simulink model "zhh"  (Simulink 7.9)
settings: Solver=FixedStepDiscrete  StartTime=0.0  StopTime=inf  FixedStep=1/256  MaxStep=1/256  RelTol=1e-3
undefined symbols (not defined in the file or in its folder): currentCFG_zhh_UB, UB
libraries: Tools x2, ScopeScaler x1, gUSBamplib x1
settings Model: Creator=gtec  LastModifiedBy=ECUSTBCI
settings OptimizationCC: InitFltsAndDblsToZero=on
settings DebuggingCC: MultiTaskCondExecSysMsg=none  FcnCallInpInsideContextMsg=Use local settings  FrameProcessingCompatibilityMsg=error  StrictBusMsg=Warning
settings GRTTargetCC: CombineOutputUpdateFcns=off  GRTInterface=on

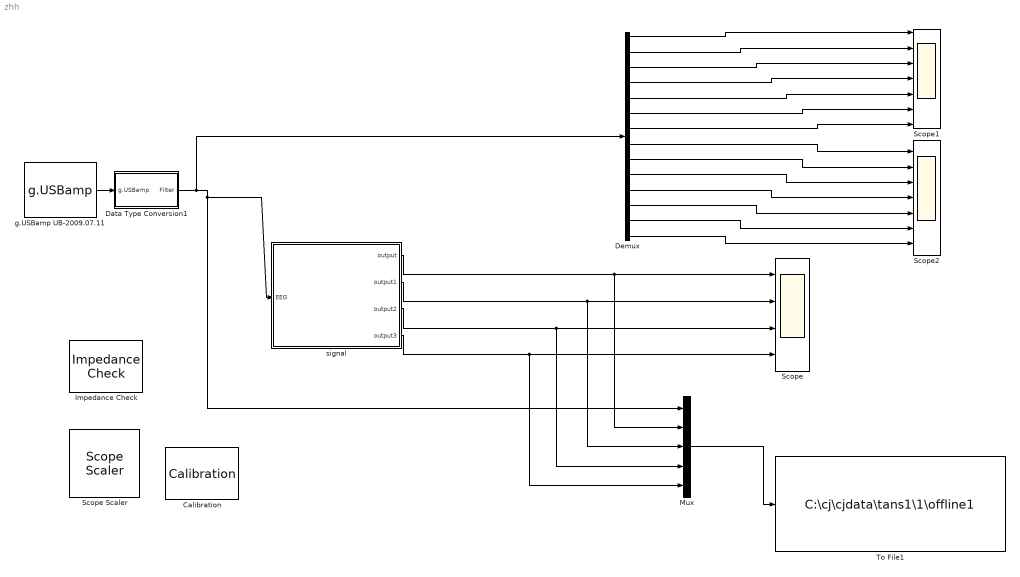
== system zhh ==
  Calibration : Tools/Calibration  SystemSampleTime=-1
  Data Type Conversion1 : Subsystem
  Demux : Demux  Outputs=14
  Impedance Check : Tools/Impedance Check  SystemSampleTime=-1
  Mux : Mux  Inputs=5
  Scope : Scope  NumInputPorts=4
      settings: TimeRange=10  YMin=9.5~9.5~9.5~9.5  YMax=10.5~10.5~10.5~10.5
  Scope Scaler : ScopeScaler/Scope Scaler  SystemSampleTime=-1
  Scope1 : Scope  NumInputPorts=7
      settings: TickLabels=off  TimeRange=10  YMin=-50~-50~-50~-50~-50~-50~-50  YMax=50~50~50~50~50~50~50  SampleTime=1/256
  Scope2 : Scope  NumInputPorts=7
      settings: TickLabels=off  TimeRange=10  YMin=-50~-50~-50~-50~-50~-50~-50  YMax=50~50~50~50~50~50~50  SaveName=ScopeData2  SampleTime=1/256
  To File1 : ToFile  Filename=C:\cj\cjdata\tans1\1\offline1  MatrixName=y
  g.USBamp UB-2009.07.11 : gUSBamplib/g.USBamp  Priority=2  cfg=currentCFG_zhh_UB-2009.07.11.cfg  snr=UB-2009.07.11
  signal : Subsystem  mask{host='192.168.1.3;192.168.1.103', socket='50000;31500', NumCustomCmds=12, ISI=500, SimNumTrials=20, ResetSpellerPeriod=300, PausePeriod=500, SampleRate=256, Determination=1, channels=14, selectchannles=[1:14], BaseAver=2, rep=2, targetp=[1 2 3 4 5 99 99 99 14 15 16 17 18 99 99 99 31 32 33 34 35 99 99 99 99 99  ], starget=1, traintime=3}
      mask prompts: host "P300host"; socket "P300socket"; NumCustomCmds "P300NumCustomCmds"; ISI "P300ISI"; SimNumTrials "P300SimNumTrials"; ResetSpellerPeriod "P300ResetSpellerPeriod"; PausePeriod "P300PausePeriod"; SampleRate "P300SampleRate"; Determination "P300Determination(classfier,yes,no)"; channels "Channles"; selectchannles "select Channels"; BaseAver "P300BaseAverage"; rep "P300reptimes"; targetp "P300target"; starget "s-target"
      mask Display:
      | image(imread('C:\tools\gtec\SSVEPP300_NET\SSVEP_MODEL2.tif'))
      | port_label('output', 1, 'flash')
      | port_label('output', 2, 'trial')
      | port_label('input', 1, 'EEG')
  wires:
  Data Type Conversion1/1(Filter) -> Mux/1, signal/1(EEG), Demux/1
  Mux/1 -> To File1/1
  signal/1(output) -> Scope/1, Mux/2
  signal/2(output1) -> Scope/2, Mux/3
  signal/3(output2) -> Scope/3, Mux/4
  signal/4(output3) -> Scope/4, Mux/5
  g.USBamp UB-2009.07.11/1 -> Data Type Conversion1/1(g.USBamp)
  Demux/1 -> Scope1/1
  Demux/2 -> Scope1/2
  Demux/3 -> Scope1/3
  Demux/4 -> Scope1/4
  Demux/5 -> Scope1/5
  Demux/6 -> Scope1/6
  Demux/7 -> Scope1/7
  Demux/8 -> Scope2/1
  Demux/9 -> Scope2/2
  Demux/10 -> Scope2/3
  Demux/11 -> Scope2/4
  Demux/12 -> Scope2/5
  Demux/13 -> Scope2/6
  Demux/14 -> Scope2/7

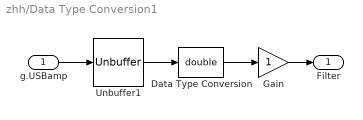
== system zhh/Data Type Conversion1 ==
  g.USBamp : Inport  Priority=1
  Data Type Conversion : DataTypeConversion  OutDataTypeStr=double
  Gain : Gain  SampleTime=1/256  SaturateOnIntegerOverflow=on  OutDataTypeStr=Inherit: Same as input  ParamDataTypeStr=Inherit: Same as input
  Unbuffer1 : Unbuffer  SampleBasedProcessing=Same as frame based
  Filter : Outport
  wires:
  Data Type Conversion/1 -> Gain/1
  Unbuffer1/1 -> Data Type Conversion/1
  Gain/1 -> Filter/1
  g.USBamp/1 -> Unbuffer1/1

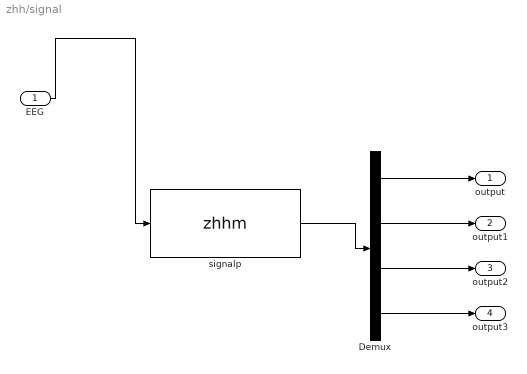
== system zhh/signal ==
  EEG : Inport
  Demux : Demux
  signalp : S-Function  FunctionName=zhhm  Parameters=host,socket,NumCustomCmds,ISI,SimNumTrials,ResetSpellerPeriod,PausePeriod,SampleRate,Determination,channels,selectchannles,BaseAver,rep,targetp,starget,traintime  EnableBusSupport=off
  output : Outport
  output1 : Outport  Port=2
  output2 : Outport  Port=3
  output3 : Outport  Port=4
  wires:
  EEG/1 -> signalp/1
  signalp/1 -> Demux/1
  Demux/1 -> output/1
  Demux/2 -> output1/1
  Demux/3 -> output2/1
  Demux/4 -> output3/1
